simulink model "MPCController"  (R2025b)
settings: Solver=VariableStepAuto  StartTime=0.0  StopTime=10  RelTol=1e-3
values from neighbouring files (symbols this model uses):
  A = [0 -56.25 0 400 1 -4.6875 0 33.3333333333 0 56.25 0 -4844.44444444 ... (16 elements, 4x4)]    [RegenVariables.mat]
  B = [0  0; -0.003125  0; 0  0; 0.0222222222222  4444.44444444]    [RegenVariables.mat]
  C = [0  1  0  0; 1  0  -1  0; 0  0  1  0]    [RegenVariables.mat]
  cs = 1500    [RegenVariables.mat]
  Cskymax = 1500    [RegenVariables.mat]
  Cskymin = 0    [RegenVariables.mat]
  D = [0  0; 0  0; 0  0]    [RegenVariables.mat]
  ks = 18000    [RegenVariables.mat]
  kt = 200000    [RegenVariables.mat]
  ms = 320    [RegenVariables.mat]
  mu = 45    [RegenVariables.mat]
  sg = 0.1    [RegenVariables.mat]
settings Model: Creator=khalidwaleed  LastModifiedBy=khalidwaleed

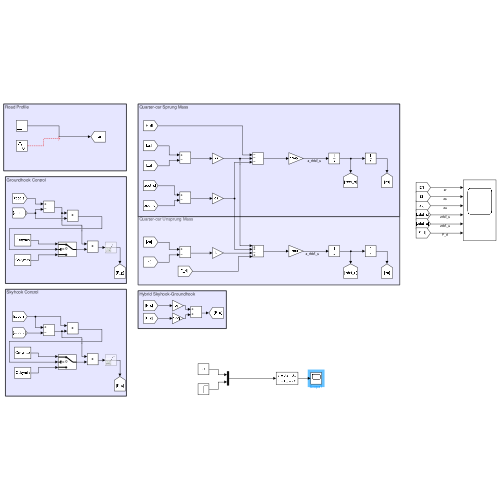
[thumbnail: Simulink's stored preview of the top-level diagram]
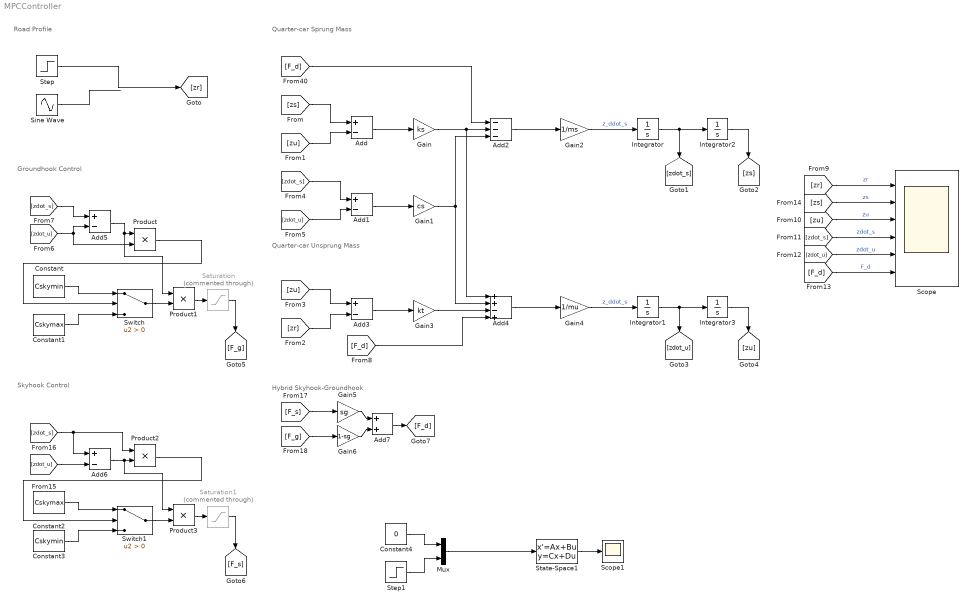
== system MPCController ==
  note: Hybrid Skyhook-Groundhook
  note: Road Profile
  note: Groundhook Control
  note: Quarter-car Sprung Mass
  note: Quarter-car Unsprung Mass
  note: Skyhook Control
  Add{,1,3,5..6} (5 alike) : Sum  Inputs=+-
  Add2 : Sum  Inputs=---
  Add4 : Sum  Inputs=++-+
  Add7 : Sum
  Constant : Constant  Value=Cskymin
  Constant1 : Constant  Value=Cskymax
  Constant2 : Constant  Value=Cskymax
  Constant3 : Constant  Value=Cskymin
  Constant4 : Constant  Value=0
  Gain : Gain  Gain=ks
  Gain1 : Gain  Gain=cs
  Gain2 : Gain  Gain=1/ms
  Gain3 : Gain  Gain=kt
  Gain4 : Gain  Gain=1/mu
  Gain5 : Gain  Gain=sg
  Gain6 : Gain  Gain=1-sg
  Integrator{,1..3} (4 alike) : Integrator
  Mux : Mux  Inputs=2
  Product{,1..3} (4 alike) : Product
  Saturation : Saturate  Commented=through  UpperLimit=2000  LowerLimit=-200
  Saturation1 : Saturate  Commented=through  UpperLimit=2000  LowerLimit=-200
  Scope : Scope  NumInputPorts=6
      settings: ActiveDisplayString=6  ActiveDisplayYMinimum=-5403.3789910212317  ActiveDisplayYMaximum=3003.5239530595863
  Scope1 : Scope
      settings: ActiveDisplayYMinimum=-3.7197551677443137  ActiveDisplayYMaximum=8.6440362489572991
  Sine Wave : Sin  Amplitude=0.02  Frequency=10  SampleTime=0
  State-Space1 : StateSpace  A=A  B=B  C=C  D=D  InitialCondition=0
  Step : Step  After=0.1  SampleTime=0
  Step1 : Step  SampleTime=0
  Switch : Switch  Criteria=u2 > Threshold  ZeroCross=off  SaturateOnIntegerOverflow=off  InputSameDT=off
  Switch1 : Switch  Criteria=u2 > Threshold  SaturateOnIntegerOverflow=off  InputSameDT=off
  wires:
  Gain2/1 -> Integrator/1  "z_ddot_s"
  [zr] -> Add3/2
  Integrator/1 -> Integrator2/1, [zdot_s]
  [zs] -> Add/1
  Add/1 -> Gain/1
  Integrator2/1 -> [zs]
  Integrator1/1 -> Integrator3/1, [zdot_u]
  [zdot_s] -> Add1/1
  Gain4/1 -> Integrator1/1  "z_ddot_s"
  Gain1/1 -> Add4/2, Add2/3
  Add2/1 -> Gain2/1
  [zu] -> Add3/1
  Add1/1 -> Gain1/1
  Gain3/1 -> Add4/3
  [zdot_u] -> Add1/2
  Add4/1 -> Gain4/1
  [F_d] -> Add2/1
  Integrator3/1 -> [zu]
  Gain/1 -> Add4/1, Add2/2
  [zu] -> Add/2
  Add3/1 -> Gain3/1
  Add5/1 -> Product1/1, Product/1
  [zdot_u] -> Product/2, Add5/2
  [zdot_s] -> Add5/1
  Product/1 -> Switch/2
  Constant/1 -> Switch/1
  Constant1/1 -> Switch/3
  Switch/1 -> Product1/2
  Step/1 -> [zr]
  Sine Wave/1 -> ?
  [F_d] -> Add4/4
  [zr] -> Scope/1  "zr"
  [F_d] -> Scope/6  "F_d"
  [zdot_u] -> Scope/5  "zdot_u"
  [zdot_s] -> Scope/4  "zdot_s"
  [zs] -> Scope/2  "zs"
  [zu] -> Scope/3  "zu"
  Product1/1 -> Saturation/1
  Saturation/1 -> [F_g]
  Saturation1/1 -> [F_s]
  [zdot_s] -> Product2/1, Add6/1
  [zdot_u] -> Add6/2
  Add6/1 -> Product3/1, Product2/2
  Product3/1 -> Saturation1/1
  Switch1/1 -> Product3/2
  Constant2/1 -> Switch1/1
  Constant3/1 -> Switch1/3
  Product2/1 -> Switch1/2
  [F_s] -> Gain5/1
  [F_g] -> Gain6/1
  Gain5/1 -> Add7/1
  Gain6/1 -> Add7/2
  Add7/1 -> [F_d]
  Mux/1 -> State-Space1/1
  State-Space1/1 -> Scope1/1
  Constant4/1 -> Mux/1
  Step1/1 -> Mux/2
